simulink model "modelo_fisico"  (Simulink 6.6)
settings: Solver=ode45  StartTime=0.0  StopTime=10.0  RelTol=1e-3
libraries: simulink x1
settings Model: Creator=spaterna  LastModifiedBy=spaterna  ExtModeAutoUpdateStatusClock=off

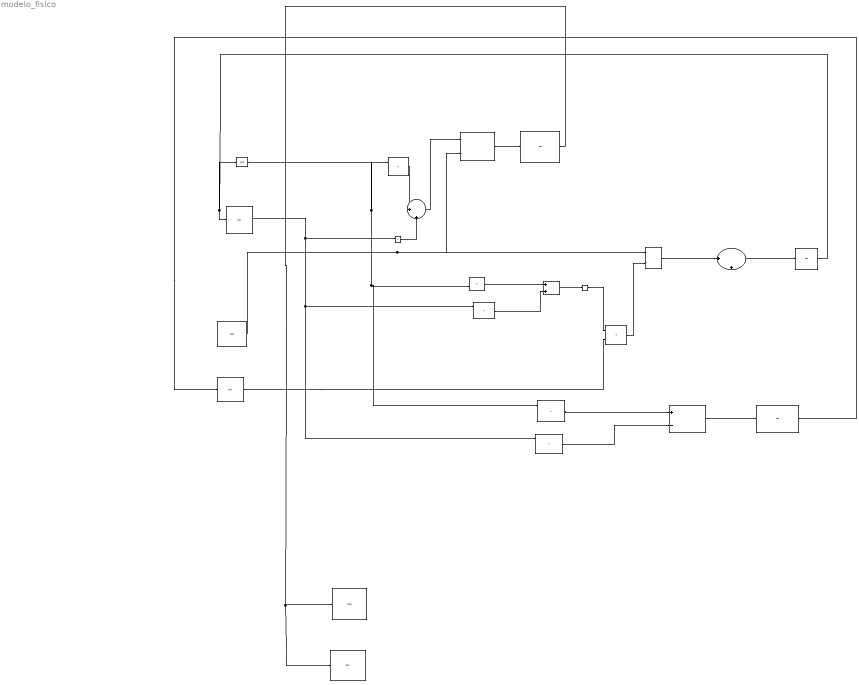
== system modelo_fisico ==
  note: cos(psi)
  note: cos(phi)
  note: sin(phi)
  note: dphi
  note: wq1
  note: phi
  Add : Sum  OutScaling=2^-10
  Divide : Product  Inputs=*/
  Divide1 : Product  Inputs=*/  OutScaling=2^-10
  Integrator : Integrator
  Integrator1 : Integrator
  Integrator2 : Integrator
  Product{,1..6} (7 alike) : Product  RndMeth=Zero
  Subtract : Sum  Inputs=+-  OutScaling=2^-10
  Sum : Sum  Inputs=|++
  Sum1 : Sum  Inputs=|++
  Trigonometric Function : Trigonometry  Operator=cos
  Trigonometric Function1 : Trigonometry
  Trigonometric Function2 : Trigonometry  Operator=cos
  Trigonometric Function3 : Trigonometry
  Trigonometric Function4 : Trigonometry
  Trigonometric Function5 : Trigonometry  Operator=cos
  Unary Minus : simulink/Math Operations/Unary Minus  DoSatur=off
  wires:
  Trigonometric Function2/1 -> Divide/2, Divide1/1
  Divide/1 -> Integrator/1  "dtheta"
  Trigonometric Function1/1 -> Product1/1, Product4/1, Product6/1  "sin(psi)"
  Trigonometric Function/1 -> Product/1, Product2/2, Product3/1
  Product/1 -> Sum/1
  ? -> Product/2  "wq3"
  ? -> Product1/2  "wq2"
  Product1/1 -> Sum/2
  Product2/1 -> Add/1
  ? -> Product2/1, Product6/2
  ? -> Product4/2, Product3/2
  Product4/1 -> Add/2
  Add/1 -> Unary Minus/1
  Product5/1 -> Divide1/2
  Divide1/1 -> Sum1/1
  ? -> Sum1/2
  Sum1/1 -> Integrator1/1  "dpsi"
  Integrator1/1 -> Trigonometric Function/1, Trigonometric Function1/1  "psi"
  Product3/1 -> Subtract/1
  Product6/1 -> Subtract/2
  Subtract/1 -> Integrator2/1
  Integrator2/1 -> Trigonometric Function3/1
  Unary Minus/1 -> Product5/1
  Trigonometric Function3/1 -> Product5/2
  Integrator/1 -> Trigonometric Function4/1, Trigonometric Function5/1  "theta"
  Sum/1 -> Divide/1
  ? -> Trigonometric Function2/1
